simulink model "gNautilusLSL"  (R2017b)
settings: Solver=FixedStepDiscrete  StartTime=0.0  StopTime=30  RelTol=1e-3  EnableMultiTasking=on
model workspace (MAT data in the model file):
  cfg_native : struct (value not decoded)
  en_add_channels = 127
  host_ip = 2130706433
  host_port = 50223
  local_ip = 2130706433
  local_port = 50224
  num_en_channels = 32
  num_samples = 8
  sample_rate = 500
  serial_number = 'NB-2017.09.08'
undefined symbols (not defined in the file or in its folder): NB
libraries: gNautilusLib x1, gtecHighspeedLib x1
settings Model: ModifiedByFormat=g.tec  Creator=g.tec medical engineering  LastModifiedBy=g.tec
settings DataIOCC: LimitDataPoints=on  SaveFormat=Array  SignalLoggingSaveFormat=ModelDataLogs
settings OptimizationCC: ExpressionDepthLimit=2147483647  InitFltsAndDblsToZero=on  LifeSpan=inf
settings DebuggingCC: UnderspecifiedInitializationDetection=Classic  MergeDetectMultiDrivingBlocksExec=none  SolverPrmCheckMsg=warning  FcnCallInpInsideContextMsg=warning  FrameProcessingCompatibilityMsg=none  StateNameClashWarn=warning  StrictBusMsg=Warning  SFUnexpectedBacktrackingDiag=warning  SFNoUnconditionalDefaultTransitionDiag=warning  SFExecutionAtInitializationDiag=none
settings HardwareCC: ProdBitPerPointer=32  ProdBitPerSizeT=32  ProdBitPerPtrDiffT=32  ProdLargestAtomicFloat=None  ProdIntDivRoundTo=Undefined  ProdEndianess=Unspecified  ProdWordSize=32  ProdHWDeviceType=32-bit Generic
settings ModelReferenceCC: PropagateSignalLabelsOutOfModel=off
settings CodeAppCC: StateflowObjectComments=on
settings GRTTargetCC: TargetLangStandard=C89/C90 (ANSI)  GeneratePreprocessorConditionals=Disable all  CombineOutputUpdateFcns=off  GRTInterface=on
settings ConfigComp: CovMetricSettings=dw  CovHtmlReporting=on  CovSaveCumulativeToWorkspaceVar=on  CovSaveSingleToWorkspaceVar=on  CovExternalEMLEnable=off

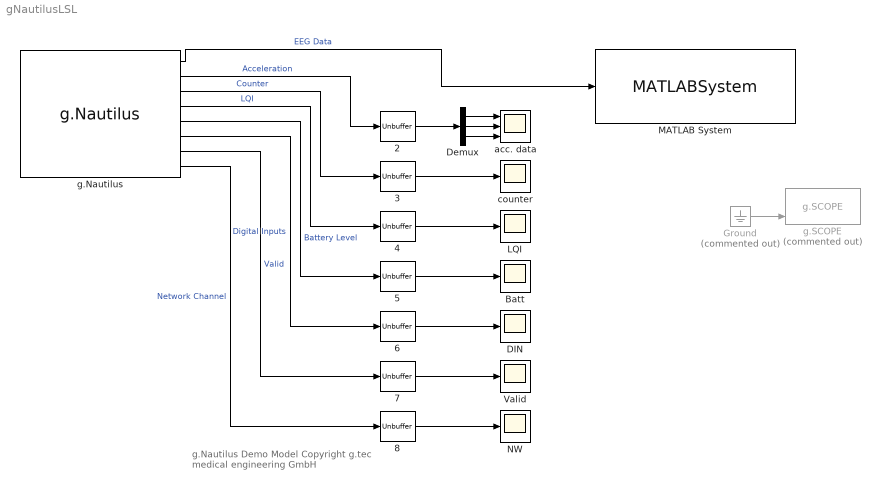
== system gNautilusLSL ==
  note: g.Nautilus Demo Model
      | Copyright g.tec medical engineering GmbH
  {2..8} (7 alike) : Unbuffer
  Batt : Scope
  DIN : Scope
  Demux : Demux  Outputs=3
  Ground : Ground  Commented=on
  LQI : Scope
  MATLAB System : MATLABSystem  System=gTecEEGExporterLSL  SimulateUsing=Code generation
      mask Type: gTecEEGExporterLSL
      mask Display:
      | disp('gTecEEGExporterLSL');
      | port_label('input',1,'chunk');
  NW : Scope
  Valid : Scope
  acc. data : Scope  NumInputPorts=3
  counter : Scope
  g.Nautilus : gNautilusLib/g.Nautilus  Tag=g.Nautilus  Description=Operates a g.Nautilus device and provides acquired data on its outputs.  sample_rate=500  local_ip=2130706433  local_port=50224  host_ip=2130706433  host_port=50223  serial_number=NB-2017.09.08  num_samples=8  num_en_channels=32  add_channels=127
      settings: SourceProductName=g.Nautilus
  g.SCOPE : gtecHighspeedLib/g.SCOPE  Commented=on
      settings: SourceProductName=g.tec Highspeed Library
  wires:
  2/1 -> Demux/1
  3/1 -> counter/1
  4/1 -> LQI/1
  g.Nautilus/2 -> 2/1  "Acceleration"
  g.Nautilus/3 -> 3/1  "Counter"
  g.Nautilus/4 -> 4/1  "LQI"
  Demux/1 -> acc. data/1
  Demux/2 -> acc. data/2
  Demux/3 -> acc. data/3
  5/1 -> Batt/1
  g.Nautilus/5 -> 5/1  "Battery Level"
  6/1 -> DIN/1
  g.Nautilus/6 -> 6/1  "Digital Inputs"
  7/1 -> Valid/1
  8/1 -> NW/1
  g.Nautilus/7 -> 7/1  "Valid"
  g.Nautilus/8 -> 8/1  "Network Channel"
  g.Nautilus/1 -> MATLAB System/1  "EEG Data"
  Ground/1 -> g.SCOPE/2
